simulink subsystem "BEV3EM"  (R2023a)
settings: Solver=VariableStepAuto  StartTime=0.0  StopTime=10.0  RelTol=1e-3
undefined symbols (not defined in the file): PlntDriveshftDamp, PlntDriveshftStiff, PlntEM1RotDamp, PlntEM1RotInertia, PlntEM2RotDamp, PlntEM2RotInertia, PlntEM3RotDamp, PlntEM3RotInertia
libraries: autolibsharedcoupling x6
settings Model: Creator=The MathWorks, Inc.  LastModifiedBy=The MathWorks, Inc.
settings OptimizationCC: ReuseModelBlockBuffer=off

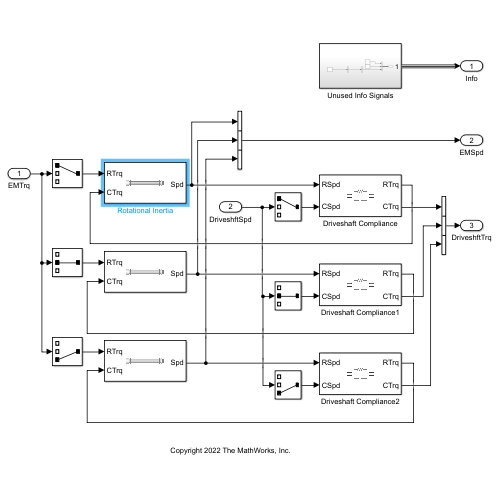
[thumbnail: Simulink's stored preview of the top-level diagram]
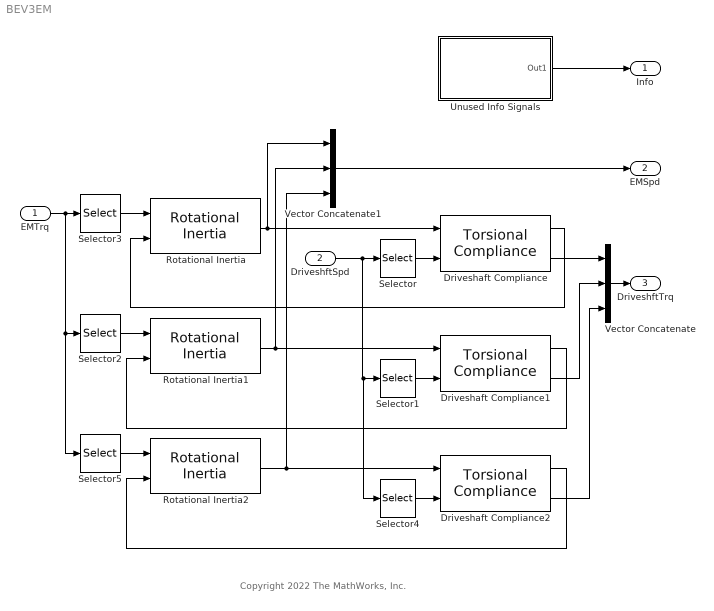
== system BEV3EM ==
  note: Copyright 2022 The MathWorks, Inc.
  EMTrq : Inport
  DriveshftSpd : Inport  Port=2
  Driveshaft Compliance : autolibsharedcoupling/Torsional Compliance  port_config=Simulink  extInfo=off  k=PlntDriveshftStiff  b=PlntDriveshftDamp  theta_o=PlntDriveshftInitDeflect  domega_o=PlntDriveshftInitVel  omega_c=PlntDriveshftDampCutoffFreq  blkID=0  aMode=1
      settings: SourceProductName=Powertrain Blockset
  Driveshaft Compliance1 : autolibsharedcoupling/Torsional Compliance  port_config=Simulink  extInfo=off  k=PlntDriveshftStiff  b=PlntDriveshftDamp  theta_o=PlntDriveshftInitDeflect  domega_o=PlntDriveshftInitVel  omega_c=PlntDriveshftDampCutoffFreq  blkID=0  aMode=1
      settings: SourceProductName=Powertrain Blockset
  Driveshaft Compliance2 : autolibsharedcoupling/Torsional Compliance  port_config=Simulink  extInfo=off  k=PlntDriveshftStiff  b=PlntDriveshftDamp  theta_o=PlntDriveshftInitDeflect  domega_o=PlntDriveshftInitVel  omega_c=PlntDriveshftDampCutoffFreq  blkID=0  aMode=1
      settings: SourceProductName=Powertrain Blockset
  Rotational Inertia : autolibsharedcoupling/Rotational Inertia  port_config=Simulink  extInfo=off  externJ=off  J=PlntEM1RotInertia  b=PlntEM1RotDamp  omega_o=PlntEM1RotInitSpd  blkID=0  aMode=1
      settings: LibrarySourceBlock=autolibcoupling/Rotational Inertia  SourceProductName=Powertrain Blockset
  Rotational Inertia1 : autolibsharedcoupling/Rotational Inertia  port_config=Simulink  extInfo=off  externJ=off  J=PlntEM2RotInertia  b=PlntEM2RotDamp  omega_o=PlntEM2RotInitSpd  blkID=0  aMode=1
      settings: LibrarySourceBlock=autolibcoupling/Rotational Inertia  SourceProductName=Powertrain Blockset
  Rotational Inertia2 : autolibsharedcoupling/Rotational Inertia  port_config=Simulink  extInfo=off  externJ=off  J=PlntEM3RotInertia  b=PlntEM3RotDamp  omega_o=PlntEM3RotInitSpd  blkID=0  aMode=1
      settings: LibrarySourceBlock=autolibcoupling/Rotational Inertia  SourceProductName=Powertrain Blockset
  Selector : Selector  InputPortWidth=3  IndexOptions=Index vector (dialog)  Indices=[1]  OutputSizes=1
  Selector1 : Selector  InputPortWidth=3  IndexOptions=Index vector (dialog)  Indices=[2]  OutputSizes=1
  Selector2 : Selector  InputPortWidth=3  IndexOptions=Index vector (dialog)  Indices=[2]  OutputSizes=1
  Selector3 : Selector  InputPortWidth=3  IndexOptions=Index vector (dialog)  Indices=[1]  OutputSizes=1
  Selector4 : Selector  InputPortWidth=3  IndexOptions=Index vector (dialog)  Indices=[3]  OutputSizes=1
  Selector5 : Selector  InputPortWidth=3  IndexOptions=Index vector (dialog)  Indices=[3]  OutputSizes=1
  Unused Info Signals : Subsystem
  Vector Concatenate : Concatenate  NumInputs=3
  Vector Concatenate1 : Concatenate  NumInputs=3
  Info : Outport  VectorParamsAs1DForOutWhenUnconnected=off  BusOutputAsStruct=on
  EMSpd : Outport  Port=2  VectorParamsAs1DForOutWhenUnconnected=off  BusOutputAsStruct=on
  DriveshftTrq : Outport  Port=3  VectorParamsAs1DForOutWhenUnconnected=off
  wires:
  Vector Concatenate1/1 -> EMSpd/1
  Selector2/1 -> Rotational Inertia1/1
  Selector3/1 -> Rotational Inertia/1
  Vector Concatenate/1 -> DriveshftTrq/1
  Driveshaft Compliance1/2 -> Vector Concatenate/2
  Selector/1 -> Driveshaft Compliance/2
  Rotational Inertia1/1 -> Driveshaft Compliance1/1, Vector Concatenate1/2
  Driveshaft Compliance/2 -> Vector Concatenate/1
  EMTrq/1 -> Selector5/1, Selector2/1, Selector3/1
  Driveshaft Compliance/1 -> Rotational Inertia/2
  Driveshaft Compliance1/1 -> Rotational Inertia1/2
  Rotational Inertia/1 -> Driveshaft Compliance/1, Vector Concatenate1/1
  Selector1/1 -> Driveshaft Compliance1/2
  Unused Info Signals/1(Out1) -> Info/1
  Selector4/1 -> Driveshaft Compliance2/2
  Driveshaft Compliance2/1 -> Rotational Inertia2/2
  DriveshftSpd/1 -> Selector4/1, Selector1/1, Selector/1
  Rotational Inertia2/1 -> Driveshaft Compliance2/1, Vector Concatenate1/3
  Driveshaft Compliance2/2 -> Vector Concatenate/3
  Selector5/1 -> Rotational Inertia2/1

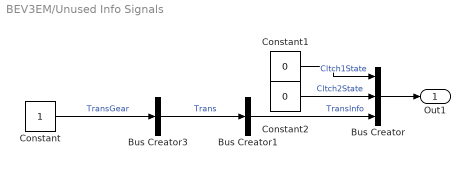
== system BEV3EM/Unused Info Signals ==
  Bus Creator : BusCreator  Inputs=3
  Bus Creator1 : BusCreator  Inputs=1
  Bus Creator3 : BusCreator  Inputs=1
  Constant : Constant  SampleTime=-1
  Constant1 : Constant  Value=0  SampleTime=-1
  Constant2 : Constant  Value=0  SampleTime=-1
  Out1 : Outport
  wires:
  Constant2/1 -> Bus Creator/2  "Cltch2State"
  Constant1/1 -> Bus Creator/1  "Cltch1State"
  Bus Creator3/1 -> Bus Creator1/1  "Trans"
  Constant/1 -> Bus Creator3/1  "TransGear"
  Bus Creator/1 -> Out1/1
  Bus Creator1/1 -> Bus Creator/3  "TransInfo"
